simulink model "TP3_3_1_3"  (R2025b)
settings: Solver=ode4  StartTime=0.0  StopTime=1  FixedStep=0.001  RelTol=1e-3
undefined symbols (not defined in the file): Bm_val, Jm_val, Kc_val, Km_val, L_val, R_val
settings Model: Creator=diegoalfonsocosta  LastModifiedBy=diegoalfonsocosta

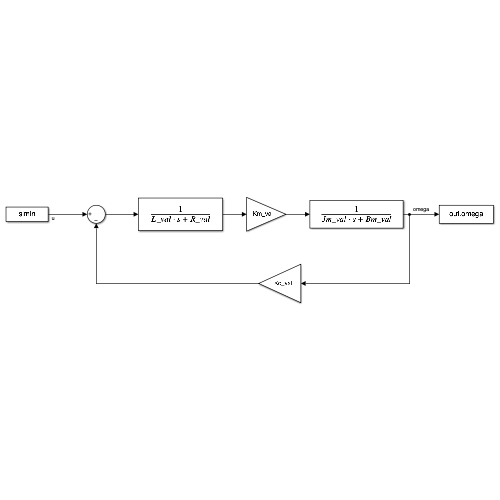
[thumbnail: Simulink's stored preview of the top-level diagram]
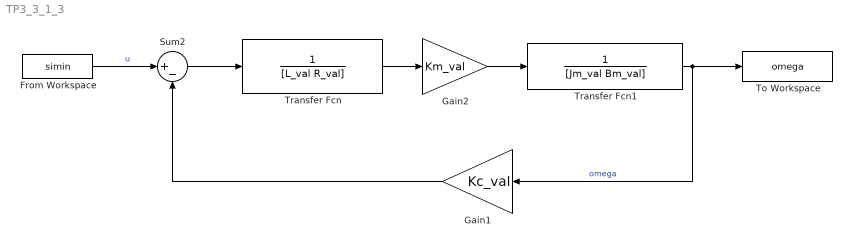
== system TP3_3_1_3 ==
  From Workspace : FromWorkspace  VariableName=simin
  Gain1 : Gain  Gain=Kc_val
  Gain2 : Gain  Gain=Km_val
  Sum2 : Sum  Inputs=|+-
  To Workspace : ToWorkspace  VariableName=omega  SaveFormat=Timeseries  SampleTime=-1
  Transfer Fcn : TransferFcn  Denominator=[L_val R_val]
  Transfer Fcn1 : TransferFcn  Numerator=1  Denominator=[Jm_val Bm_val]
  wires:
  Transfer Fcn1/1 -> Gain1/1, To Workspace/1  "omega"
  Gain1/1 -> Sum2/2
  From Workspace/1 -> Sum2/1  "u"
  Sum2/1 -> Transfer Fcn/1
  Transfer Fcn/1 -> Gain2/1
  Gain2/1 -> Transfer Fcn1/1
